simulink model "Math_Operations_1"  (R2024b)
settings: Solver=FixedStepAuto  StartTime=0.0  StopTime=10.0  RelTol=1e-3
settings Model: Creator=Minkyo  LastModifiedBy=Minkyo
settings OptimizationCC: DefaultParameterBehavior=Inlined  UseDivisionForNetSlopeComputation=on  GainParamInheritBuiltInType=on  UseFloatMulNetSlope=on  InlineInvariantSignals=on  PassReuseOutputArgsAs=Individual arguments  ZeroExternalMemoryAtStartup=off  ZeroInternalMemoryAtStartup=off  NoFixptDivByZeroProtection=on  EfficientFloat2IntCast=on  LifeSpan=1  OptimizeBlockOrder=speed  DifferentSizesBufferReuse=on  EfficientTunableParamExpr=on
settings DebuggingCC: ParameterTunabilityLossMsg=error
settings HardwareCC: ProdLongLongMode=on
settings SFSimCC: MATLABDynamicMemAlloc=off
settings RTWCC: Description=Embedded Coder  SystemTargetFile=ert.tlc  TemplateMakefile=ert_default_tmf
settings CodeAppCC: ForceParamTrailComments=on  IgnoreCustomStorageClasses=off  OperatorAnnotations=on  SimulinkDataObjDesc=on  SFDataObjDesc=on  CustomSymbolStrGlobalVar=rt$N$M  CustomSymbolStrType=$N$M  CustomSymbolStrFcn=$N$M$F  CustomSymbolStrMacro=$N$M  InsertBlockDesc=on
settings ERTTargetCC: TargetLangStandard=C99 (ISO)  GenerateSampleERTMain=on  IncludeMdlTerminateFcn=off  CombineSignalStateStructs=on  SupportAbsoluteTime=off  SupportComplex=off  SupportContinuousTime=on  ERTCustomFileTemplate=example_file_process.tlc  ERTFilePackagingFormat=CompactWithDataFile

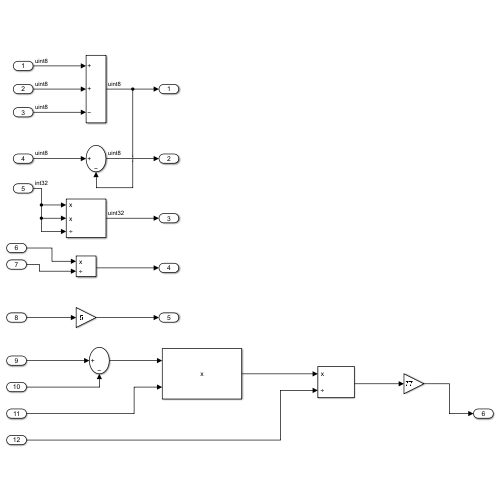
[thumbnail: Simulink's stored preview of the top-level diagram]
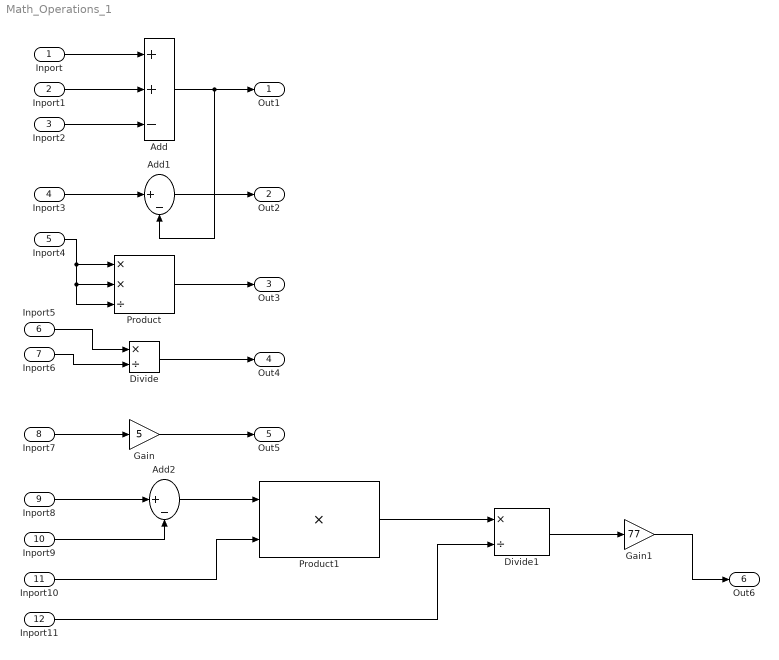
== system Math_Operations_1 ==
  Inport : Inport
  Inport1 : Inport  Port=2
  Inport2 : Inport  Port=3
  Inport3 : Inport  Port=4  OutDataTypeStr=uint8
  Inport4 : Inport  Port=5  OutDataTypeStr=int32
  Inport5 : Inport  Port=6
  Inport6 : Inport  Port=7
  Inport7 : Inport  Port=8
  Inport8 : Inport  Port=9
  Inport9 : Inport  Port=10
  Inport10 : Inport  Port=11
  Inport11 : Inport  Port=12
  Add : Sum  Inputs=++-
  Add1 : Sum  Inputs=|+-
  Add2 : Sum  Inputs=|+-
  Divide : Product  Inputs=*/
  Divide1 : Product  Inputs=*/
  Gain : Gain  Gain=5
  Gain1 : Gain  Gain=77
  Product : Product  Inputs=**/  OutDataTypeStr=uint32
  Product1 : Product
  Out1 : Outport
  Out2 : Outport  Port=2
  Out3 : Outport  Port=3
  Out4 : Outport  Port=4
  Out5 : Outport  Port=5
  Out6 : Outport  Port=6
  wires:
  Inport/1 -> Add/1
  Inport1/1 -> Add/2
  Inport2/1 -> Add/3
  Add/1 -> Add1/2, Out1/1
  Inport3/1 -> Add1/1
  Add1/1 -> Out2/1
  Product/1 -> Out3/1
  Inport4/1 -> Product/1, Product/2, Product/3
  Divide/1 -> Out4/1
  Inport5/1 -> Divide/1
  Inport6/1 -> Divide/2
  Inport7/1 -> Gain/1
  Gain/1 -> Out5/1
  Inport8/1 -> Add2/1
  Inport9/1 -> Add2/2
  Add2/1 -> Product1/1
  Inport10/1 -> Product1/2
  Product1/1 -> Divide1/1
  Inport11/1 -> Divide1/2
  Divide1/1 -> Gain1/1
  Gain1/1 -> Out6/1
